simulink model "differential_drive_base_robot_voltage_loop"  (R2015b)
settings: Solver=VariableStepAuto  StartTime=0.0  StopTime=10  RelTol=1e-3
values from neighbouring files (symbols this model uses):
  B = 0.1    [andbot1dot2_modeling_param.m]    (also in andbot1dot2_param.m)
  J = 0.1    [andbot1dot2_modeling_param.m]    (also in andbot1dot2_param.m)
  ke = 0.31    [andbot1dot2_modeling_param.m]    (also in andbot1dot2_param.m)
  kt = 0.01    [andbot1dot2_modeling_param.m]    (also in andbot1dot2_param.m)
  l = 0.41367 / 2    (= 0.206835)    [andbot1dot2_modeling_param.m]    (also in andbot1dot2_param.m)
  m = 18.8    [andbot1dot2_modeling_param.m]    (also in andbot1dot2_param.m)
  r = 0.085    [andbot1dot2_modeling_param.m]    (also in andbot1dot2_param.m)
  R = 0.02    [andbot1dot2_modeling_param.m]    (also in andbot1dot2_param.m)
settings Model: Creator=shangwei  LastModifiedBy=root

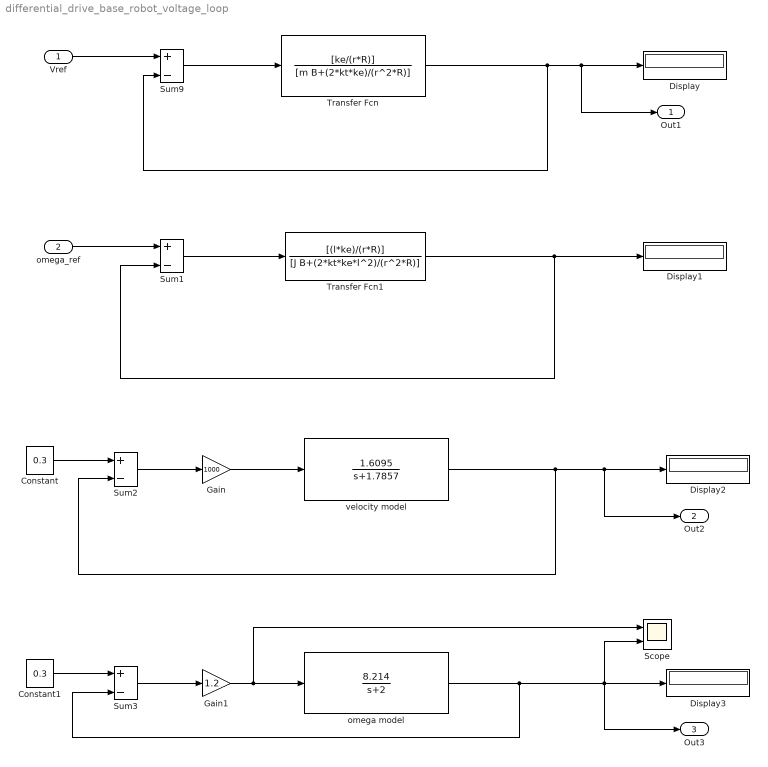
== system differential_drive_base_robot_voltage_loop ==
  Vref : Inport
  omega_ref : Inport  Port=2
  Constant : Constant  Value=0.3
  Constant1 : Constant  Value=0.3
  Display{,1..3} (4 alike) : Display
  Gain : Gain  Gain=1000
  Gain1 : Gain  Gain=1.2
  Scope : Scope  NumInputPorts=2
  Sum{1..3,9} (4 alike) : Sum  Inputs=+-
  Transfer Fcn : TransferFcn  Numerator=[ke/(r*R)]  Denominator=[m B+(2*kt*ke)/(r^2*R)]
  Transfer Fcn1 : TransferFcn  Numerator=[(l*ke)/(r*R)]  Denominator=[J B+(2*kt*ke*l^2)/(r^2*R)]
  omega model : TransferFcn  Numerator=[8.214]  Denominator=[1 2]
  velocity model : TransferFcn  Numerator=[1.6095]  Denominator=[1 1.7857]
  Out1 : Outport
  Out2 : Outport  Port=2
  Out3 : Outport  Port=3
  wires:
  Sum9/1 -> Transfer Fcn/1
  Transfer Fcn/1 -> Sum9/2, Out1/1, Display/1
  Vref/1 -> Sum9/1
  Sum1/1 -> Transfer Fcn1/1
  omega_ref/1 -> Sum1/1
  Transfer Fcn1/1 -> Sum1/2, Display1/1
  Sum2/1 -> Gain/1
  velocity model/1 -> Sum2/2, Display2/1, Out2/1
  Constant/1 -> Sum2/1
  Gain/1 -> velocity model/1
  Sum3/1 -> Gain1/1
  omega model/1 -> Sum3/2, Scope/2, Out3/1, Display3/1
  Constant1/1 -> Sum3/1
  Gain1/1 -> Scope/1, omega model/1
